simulink library "fms"  (Simulink 8.1)
settings: Solver=ode1  StartTime=0.0  StopTime=Inf  FixedStep=0.001  RelTol=1e-3
PostLoadFcn:
  | , if any(exist('dsrtsu_mdlpostloadfcn', 'file') == [2, 3, 6]), try dsrtsu_mdlpostloadfcn('Execute', bdroot); catch fprintf('Error in PostLoadFcn (dsrtsu_mdlpostloadfcn) for model "%s":\n %s\n', bdroot, lasterr); end, end,
undefined symbols (not defined in the file or in its folder): KIFO_FCWExistProbLimit_num, ZERO_INT
settings Model: DSRTSU_INTERNAL_RTI_VER=450  DSRTSU_INTERNAL_RTI_TYPE=rti1401  RTICANMMDATA=struct('GeneralSetupData',struct('modelroot','D:\ELN150201_TAIWAN\trunk\AdasDragon\software\sw_development\arch\app\ifo','generalsettings',struct('filesettings',struct('destfolder',struct('Name','RTICANMM_FILES','Check',1),'buildfolder',struct('Name','.','Check',1),'AbsDestfolder',struct('Name','D:\ELN150201_TAIWAN\trunk\AdasDragon\software\sw_development\arch\app\ifo\RTICANMM_FILES'),'AbsBuildfolder',struct('Name','D:\ELN150201_TAIWAN\trunk\AdasDragon\software\sw_development\arch\app\ifo'))),'options',struct('addpaths',1,'rmpaths',1,'addtrcexclusion',logical(1),'cannavigator',struct('checkmonitoring',0),'show_usrtrc',0,'use_usrtrc',0),'advanced',struct('options',[1 1 1 1 1 1 1 1 1 1 1 1 1 1 1 1 1 1 1 1 1 1 1 1 1 1 1 1 1 1 1 1 1 1 1 1 1 1 1 1 1 1 1 1 1 1 1 1 1 1 1 1 1 1 1 1 1 1 1 1 1 1 1 1 1 1 1 1 1 1 1 1 1 1 1 1 1 1 1 1 1 1 1 1 1 1 1 1 1 1 1 1 1 1 1 1 1 1 1 1]),'MPSetup',{{}},'modelname','fms','block','fms'))  DSRTSU_INTERNAL_RTIFPGA=40  Creator=tescamilla  LastModifiedBy=AT015555

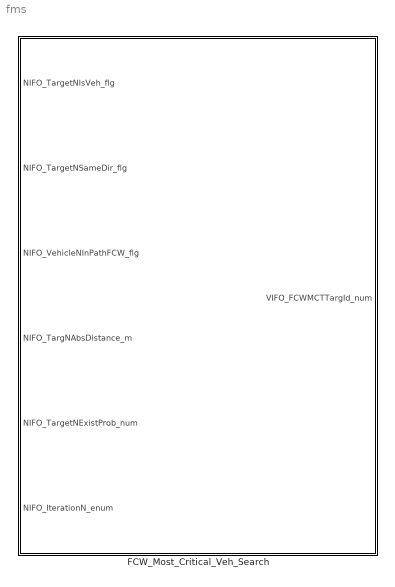
== system fms ==
  FCW_Most_Critical_Veh_Search : Subsystem

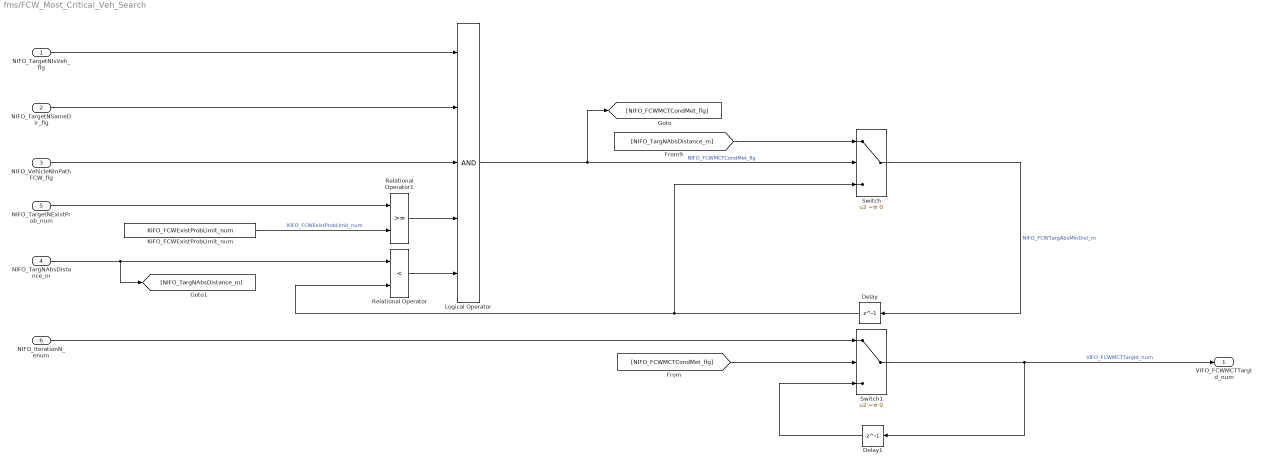
== system fms/FCW_Most_Critical_Veh_Search ==
  NIFO_TargetNIsVeh_flg : Inport
  NIFO_TargetNSameDir_flg : Inport  Port=2
  NIFO_VehicleNInPathFCW_flg : Inport  Port=3
  NIFO_TargNAbsDistance_m : Inport  Port=4
  NIFO_TargetNExistProb_num : Inport  Port=5
  NIFO_IterationN_enum : Inport  Port=6
  Delay : Delay  DelayLength=1  InitialCondition=1000
  Delay1 : Delay  DelayLength=1  InitialCondition=ZERO_INT
  KIFO_FCWExistProbLimit_num : Constant  Value=KIFO_FCWExistProbLimit_num
  Logical Operator : Logic  Inputs=5  AllPortsSameDT=off  OutDataTypeStr=boolean
  Relational Operator : RelationalOperator  Operator=<  OutDataTypeStr=boolean
  Relational Operator1 : RelationalOperator  OutDataTypeStr=boolean
  Switch : Switch  Criteria=u2 ~= 0
  Switch1 : Switch  Criteria=u2 ~= 0
  VIFO_FCWMCTTargId_num : Outport
  wires:
  NIFO_TargNAbsDistance_m/1 -> [NIFO_TargNAbsDistance_m], Relational Operator/1
  NIFO_TargetNSameDir_flg/1 -> Logical Operator/2
  NIFO_TargetNIsVeh_flg/1 -> Logical Operator/1
  Relational Operator/1 -> Logical Operator/5
  Delay/1 -> Relational Operator/2, Switch/3
  Delay1/1 -> Switch1/3
  Logical Operator/1 -> Switch/2, [NIFO_FCWMCTCondMet_flg]  "NIFO_FCWMCTCondMet_flg"
  [NIFO_TargNAbsDistance_m] -> Switch/1
  Switch1/1 -> VIFO_FCWMCTTargId_num/1, Delay1/1  "VIFO_FCWMCTTargId_num"
  NIFO_VehicleNInPathFCW_flg/1 -> Logical Operator/3
  Switch/1 -> Delay/1  "NIFO_FCWTargAbsMinDist_m"
  [NIFO_FCWMCTCondMet_flg] -> Switch1/2
  NIFO_IterationN_enum/1 -> Switch1/1
  NIFO_TargetNExistProb_num/1 -> Relational Operator1/1
  KIFO_FCWExistProbLimit_num/1 -> Relational Operator1/2  "KIFO_FCWExistProbLimit_num"
  Relational Operator1/1 -> Logical Operator/4
